simulink model "simplebc_tl"  (Simulink 7.3)
settings: Solver=FixedStepDiscrete  SolverMode=SingleTasking  StartTime=0.0  StopTime=400  FixedStep=tsample  RelTol=1e-3
PreLoadFcn:
  | if exist('tl_preloadfcn','file'), tl_preloadfcn(gcs,101); end
PostLoadFcn:
  | if exist('tl_postloadfcn','file'), tl_postloadfcn(gcs,101); end
InitFcn:
  | if exist('tlds_init','file'), tlds_init(gcs); end
StartFcn:
  | if exist('tlds_start','file'), tlds_start(gcs); end
StopFcn:
  | if exist('tlds_stop','file'), tlds_stop(gcs); end
values from neighbouring files (symbols this model uses):
  fs_max = 4000    [simplebc_mdl.m]
  fs_min = 1000    [simplebc_mdl.m]
  maxcnt_heating = 10    [simplebc_mdl.m]
  maxcnt_ign = 3    [simplebc_mdl.m]
  maxcnt_preign = 2    [simplebc_mdl.m]
  maxcnt_prev1 = 3    [simplebc_mdl.m]
  maxcnt_prev2 = 8    [simplebc_mdl.m]
  maxcnt_standby = 10    [simplebc_mdl.m]
  srinp_resptime = 2    [simplebc_mdl.m]
  srinp_testcycletime = 3    [simplebc_mdl.m]
  sroutp_resptime = 2    [simplebc_mdl.m]
  sroutp_testcycletime = 3    [simplebc_mdl.m]
  tsample = 0.1    [simplebc_mdl.m]
libraries: tllib x6, simulink x6
(part 1 of 2)
PreSaveFcn:
  | if exist('tl_presavefcn','file'), tl_presavefcn(gcs); end
settings Model: DS_PROJECTFILE=simplebc.dd  TL_MAIN_DATA={'#advcodeopt',0,'frameopt',{'mexargs',''},'logopt',{'plotinterval',0.1,'globalloggingmode',4},'date',734178.39644840278}  TL_MODEL_COMMENT=Type in your documentation HERE  TLRevision=101  Creator=alexh  LastModifiedBy=qa_user  BufferReuse=off
settings OptimizationCC: BlockReduction=off  BooleanDataType=off  InlineInvariantSignals=on  OptimizeBlockIOStorage=off  BufferReuse=off  ExpressionFolding=off  LocalBlockOutputs=off  InitFltsAndDblsToZero=on
settings DebuggingCC: SaveWithParameterizedLinksMsg=none  SignalResolutionControl=TryResolveAllWithWarning  SolverPrmCheckMsg=none  MultiTaskDSMMsg=warning  MultiTaskCondExecSysMsg=none  StrictBusMsg=ErrorLevel1
settings HardwareCC: TargetUnknown=on
settings RTWCC: IncludeERTFirstTime=on
settings GRTTargetCC: TargetFcnLib=ansi_tfl_tmw.mat  ModelReferenceCompliant=off  MatFileLogging=off

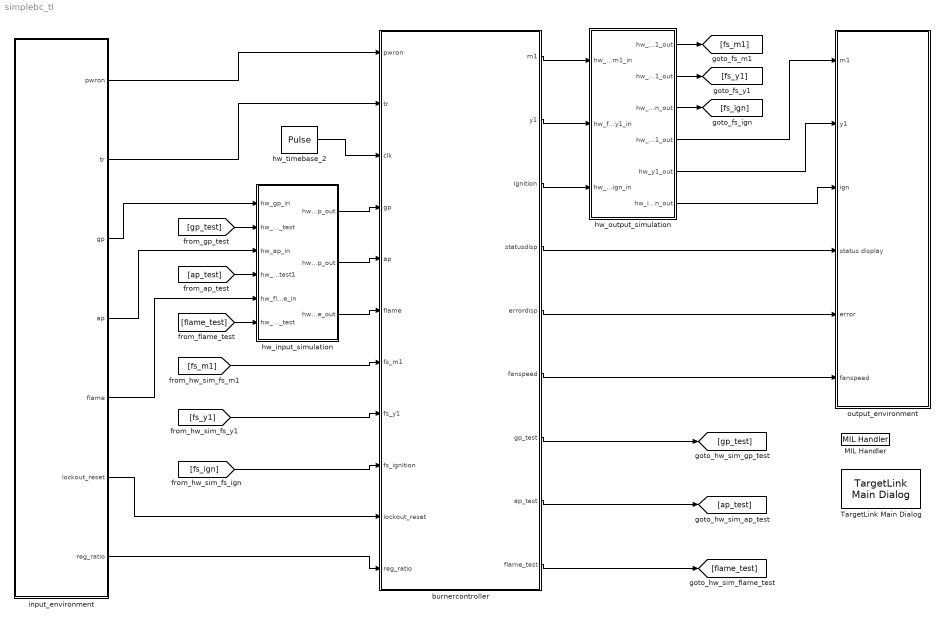
== system simplebc_tl ==
  MIL Handler : tllib/MIL Handler  data={'date',734178.39643827546}
  TargetLink Main Dialog : tllib/TargetLink Main Dialog  SystemSampleTime=-1
  burnercontroller : Subsystem  Tag=TargetLink Simulation Frame
      settings: CopyFcn=if exist('tl_copyfcn','file'), tl_copyfcn(gcbh); end  NameChangeFcn=if exist('tl_framenamechangefcn','file'), tl_framenamechangefcn(gcbh); end
      settings: OpenFcn=|
      | if exist('open_tlsubsystem','file')
      |    open_tlsubsystem(gcbh);
      | else
      |    tlsubsystem = ...
      |       find_system(gcb, ...
      |       'LookUnderMasks','on', ...
      |       'FollowLinks','on', ...
      |       'Tag','MIL Subsystem');
      |    open_system(tlsubsystem);
      | end
      mask Type: TL_SimFrame
      mask Display: disp('TargetLink\nModel-\nin-the-loop\nmode')
  hw_input_simulation : Subsystem
  hw_output_simulation : Subsystem
  hw_timebase_2 : DiscretePulseGenerator  PulseType=Time based  Amplitude=1  Period=tsample*2  PulseWidth=50  PhaseDelay=0  SampleTime=1
  input_environment : Subsystem
  output_environment : Subsystem
  wires:
  hw_input_simulation/1(hw_gp_out) -> burnercontroller/4(gp)
  input_environment/3(gp) -> hw_input_simulation/1(hw_gp_in)
  hw_input_simulation/2(hw_ap_out) -> burnercontroller/5(ap)
  hw_input_simulation/3(hw_flame_out) -> burnercontroller/6(flame)
  input_environment/4(ap) -> hw_input_simulation/3(hw_ap_in)
  input_environment/5(flame) -> hw_input_simulation/5(hw_flame_in)
  burnercontroller/8(ap_test) -> [ap_test]
  burnercontroller/9(flame_test) -> [flame_test]
  [flame_test] -> hw_input_simulation/6(hw_flame_test)
  [ap_test] -> hw_input_simulation/4(hw_ap_test1)
  [gp_test] -> hw_input_simulation/2(hw_gp_test)
  input_environment/6(lockout_reset) -> burnercontroller/10(lockout_reset)
  burnercontroller/1(m1) -> hw_output_simulation/1(hw_fs_m1_in)
  burnercontroller/2(y1) -> hw_output_simulation/2(hw_fs_y1_in)
  burnercontroller/3(ignition) -> hw_output_simulation/3(hw_fs_ign_in)
  hw_output_simulation/6(hw_ign_out) -> output_environment/3(ign)
  hw_output_simulation/3(hw_fs_ign_out) -> [fs_ign]
  hw_output_simulation/1(hw_fs_m1_out) -> [fs_m1]
  hw_output_simulation/2(hw_fs_y1_out) -> [fs_y1]
  [fs_ign] -> burnercontroller/9(fs_ignition)
  [fs_y1] -> burnercontroller/8(fs_y1)
  [fs_m1] -> burnercontroller/7(fs_m1)
  burnercontroller/4(statusdisp) -> output_environment/4(status display)
  burnercontroller/5(errordisp) -> output_environment/5(error)
  hw_output_simulation/4(hw_m1_out) -> output_environment/1(m1)
  hw_output_simulation/5(hw_y1_out) -> output_environment/2(y1)
  input_environment/7(reg_ratio) -> burnercontroller/11(reg_ratio)
  input_environment/1(pwron) -> burnercontroller/1(pwron)
  input_environment/2(tr) -> burnercontroller/2(tr)
  hw_timebase_2/1 -> burnercontroller/3(clk)
  burnercontroller/7(gp_test) -> [gp_test]
  burnercontroller/6(fanspeed) -> output_environment/6(fanspeed)

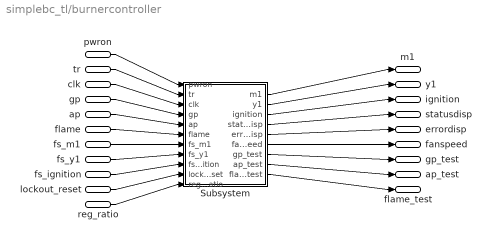
== system simplebc_tl/burnercontroller ==
  pwron : Inport  OutDataType=sfix(16)  OutScaling=2^0
  tr : Inport  Port=2  OutDataType=sfix(16)  OutScaling=2^0
  clk : Inport  Port=3  OutDataType=sfix(16)  OutScaling=2^0
  gp : Inport  Port=4  OutDataType=sfix(16)  OutScaling=2^0
  ap : Inport  Port=5  OutDataType=sfix(16)  OutScaling=2^0
  flame : Inport  Port=6  OutDataType=sfix(16)  OutScaling=2^0
  fs_m1 : Inport  Port=7  SampleTime=tsample  OutDataType=sfix(16)  OutScaling=2^0
  fs_y1 : Inport  Port=8  SampleTime=tsample  OutDataType=sfix(16)  OutScaling=2^0
  fs_ignition : Inport  Port=9  SampleTime=tsample  OutDataType=sfix(16)  OutScaling=2^0
  lockout_reset : Inport  Port=10  OutDataType=sfix(16)  OutScaling=2^0
  reg_ratio : Inport  Port=11  OutDataType=sfix(16)  OutScaling=2^0
  Subsystem : Subsystem  Tag=struct('sfcnName','burnercontroller_sf','subFunction','','srcSubsystem','')
      settings: OpenFcn=warndlg(get_param(gcb,'MaskHelp'),'Serious Warning');
      mask Type: TL_Enable
      mask Help: This subsystem keeps the TargetLink subsystem (subsystem with TargetLink blocks for production code generation), and is needed for the TargetLink simulation frame to work properly. DO NOT DELETE OR MODIFY IT!
  m1 : Outport  OutDataType=sfix(16)  OutScaling=2^0
  y1 : Outport  Port=2  OutDataType=sfix(16)  OutScaling=2^0
  ignition : Outport  Port=3  OutDataType=sfix(16)  OutScaling=2^0
  statusdisp : Outport  Port=4  OutDataType=sfix(16)  OutScaling=2^0
  errordisp : Outport  Port=5  OutDataType=sfix(16)  OutScaling=2^0
  fanspeed : Outport  Port=6  OutDataType=sfix(16)  OutScaling=2^0
  gp_test : Outport  Port=7  OutDataType=sfix(16)  OutScaling=2^0
  ap_test : Outport  Port=8  OutDataType=sfix(16)  OutScaling=2^0
  flame_test : Outport  Port=9  OutDataType=sfix(16)  OutScaling=2^0
  wires:
  pwron/1 -> Subsystem/1(pwron)
  tr/1 -> Subsystem/2(tr)
  clk/1 -> Subsystem/3(clk)
  gp/1 -> Subsystem/4(gp)
  ap/1 -> Subsystem/5(ap)
  flame/1 -> Subsystem/6(flame)
  fs_m1/1 -> Subsystem/7(fs_m1)
  fs_y1/1 -> Subsystem/8(fs_y1)
  fs_ignition/1 -> Subsystem/9(fs_ignition)
  lockout_reset/1 -> Subsystem/10(lockout_reset)
  reg_ratio/1 -> Subsystem/11(reg_ratio)
  Subsystem/1(m1) -> m1/1
  Subsystem/2(y1) -> y1/1
  Subsystem/3(ignition) -> ignition/1
  Subsystem/4(statusdisp) -> statusdisp/1
  Subsystem/5(errordisp) -> errordisp/1
  Subsystem/6(fanspeed) -> fanspeed/1
  Subsystem/7(gp_test) -> gp_test/1
  Subsystem/8(ap_test) -> ap_test/1
  Subsystem/9(flame_test) -> flame_test/1

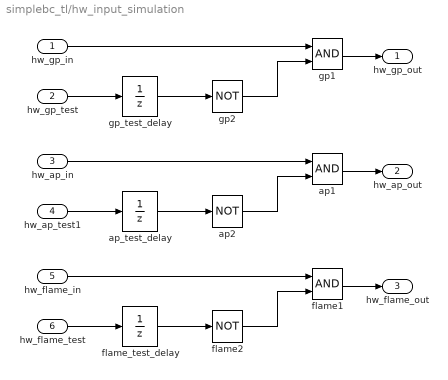
== system simplebc_tl/hw_input_simulation ==
  hw_gp_in : Inport  OutDataType=sfix(16)  OutScaling=2^0
  hw_gp_test : Inport  Port=2  OutDataType=sfix(16)  OutScaling=2^0
  hw_ap_in : Inport  Port=3  OutDataType=sfix(16)  OutScaling=2^0
  hw_ap_test1 : Inport  Port=4  OutDataType=sfix(16)  OutScaling=2^0
  hw_flame_in : Inport  Port=5  OutDataType=sfix(16)  OutScaling=2^0
  hw_flame_test : Inport  Port=6  OutDataType=sfix(16)  OutScaling=2^0
  ap1 : Logic
  ap2 : Logic  Operator=NOT  Inputs=1
  ap_test_delay : UnitDelay  SampleTime=tsample*2
  flame1 : Logic
  flame2 : Logic  Operator=NOT  Inputs=1
  flame_test_delay : UnitDelay  SampleTime=tsample*2
  gp1 : Logic
  gp2 : Logic  Operator=NOT  Inputs=1
  gp_test_delay : UnitDelay  SampleTime=tsample*2
  hw_gp_out : Outport  OutDataType=sfix(16)  OutScaling=2^0
  hw_ap_out : Outport  Port=2  OutDataType=sfix(16)  OutScaling=2^0
  hw_flame_out : Outport  Port=3  OutDataType=sfix(16)  OutScaling=2^0
  wires:
  gp2/1 -> gp1/2
  gp_test_delay/1 -> gp2/1
  hw_gp_test/1 -> gp_test_delay/1
  hw_gp_in/1 -> gp1/1
  gp1/1 -> hw_gp_out/1
  ap2/1 -> ap1/2
  ap_test_delay/1 -> ap2/1
  hw_ap_test1/1 -> ap_test_delay/1
  hw_ap_in/1 -> ap1/1
  ap1/1 -> hw_ap_out/1
  flame2/1 -> flame1/2
  flame_test_delay/1 -> flame2/1
  hw_flame_test/1 -> flame_test_delay/1
  hw_flame_in/1 -> flame1/1
  flame1/1 -> hw_flame_out/1

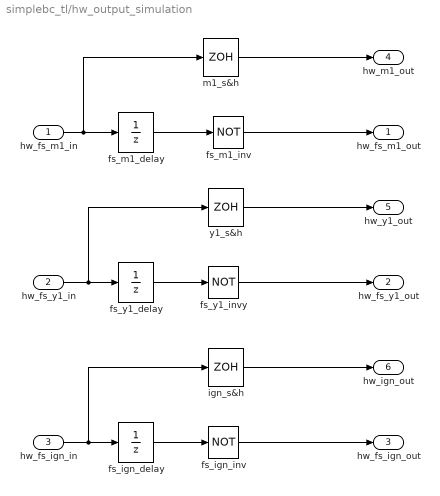
== system simplebc_tl/hw_output_simulation ==
  hw_fs_m1_in : Inport  OutDataType=sfix(16)  OutScaling=2^0
  hw_fs_y1_in : Inport  Port=2  OutDataType=sfix(16)  OutScaling=2^0
  hw_fs_ign_in : Inport  Port=3  OutDataType=sfix(16)  OutScaling=2^0
  fs_ign_delay : UnitDelay  SampleTime=tsample*2
  fs_ign_inv : Logic  Operator=NOT  Inputs=1
  fs_m1_delay : UnitDelay  SampleTime=tsample*2
  fs_m1_inv : Logic  Operator=NOT  Inputs=1
  fs_y1_delay : UnitDelay  SampleTime=tsample*2
  fs_y1_invy : Logic  Operator=NOT  Inputs=1
  ign_s&h : ZeroOrderHold  SampleTime=tsample*(sroutp_testcycletime+sroutp_resptime)
  m1_s&h : ZeroOrderHold  SampleTime=tsample*(sroutp_testcycletime+sroutp_resptime)
  y1_s&h : ZeroOrderHold  SampleTime=tsample*(sroutp_testcycletime+sroutp_resptime)
  hw_fs_m1_out : Outport  OutDataType=sfix(16)  OutScaling=2^0
  hw_fs_y1_out : Outport  Port=2  OutDataType=sfix(16)  OutScaling=2^0
  hw_fs_ign_out : Outport  Port=3  OutDataType=sfix(16)  OutScaling=2^0
  hw_m1_out : Outport  Port=4  OutDataType=sfix(16)  OutScaling=2^0
  hw_y1_out : Outport  Port=5  OutDataType=sfix(16)  OutScaling=2^0
  hw_ign_out : Outport  Port=6  OutDataType=sfix(16)  OutScaling=2^0
  wires:
  fs_m1_inv/1 -> hw_fs_m1_out/1
  hw_fs_m1_in/1 -> fs_m1_delay/1, m1_s&h/1
  m1_s&h/1 -> hw_m1_out/1
  fs_y1_delay/1 -> fs_y1_invy/1
  fs_y1_invy/1 -> hw_fs_y1_out/1
  hw_fs_y1_in/1 -> fs_y1_delay/1, y1_s&h/1
  y1_s&h/1 -> hw_y1_out/1
  fs_ign_delay/1 -> fs_ign_inv/1
  fs_ign_inv/1 -> hw_fs_ign_out/1
  hw_fs_ign_in/1 -> fs_ign_delay/1, ign_s&h/1
  ign_s&h/1 -> hw_ign_out/1
  fs_m1_delay/1 -> fs_m1_inv/1

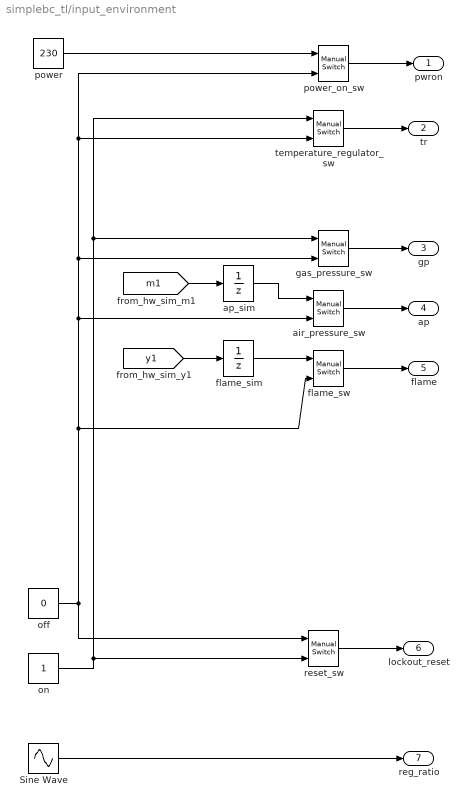
== system simplebc_tl/input_environment ==
  Sine Wave : Sin  Amplitude=50  Bias=50  Frequency=0.01  Phase=0  Samples=10  SampleTime=0  Offset=0
  air_pressure_sw : simulink/Signal Routing/Manual Switch  SystemSampleTime=-1  sw=1  action=0  varsize=off
  ap_sim : UnitDelay  SampleTime=tsample*10
  flame_sim : UnitDelay  SampleTime=tsample*10
  flame_sw : simulink/Signal Routing/Manual Switch  SystemSampleTime=-1  sw=1  action=0  varsize=off
  gas_pressure_sw : simulink/Signal Routing/Manual Switch  SystemSampleTime=-1  sw=1  action=0  varsize=off
  off : Constant  Value=0  OutDataType=sfix(16)  OutScaling=2^0
  on : Constant  OutDataType=sfix(16)  OutScaling=2^0
  power : Constant  Value=230  OutDataType=sfix(16)  OutScaling=2^0
  power_on_sw : simulink/Signal Routing/Manual Switch  SystemSampleTime=-1  sw=1  action=0  varsize=off
  reset_sw : simulink/Signal Routing/Manual Switch  SystemSampleTime=-1  sw=1  action=0  varsize=off
  temperature_regulator_sw : simulink/Signal Routing/Manual Switch  SystemSampleTime=-1  sw=1  action=0  varsize=off
  pwron : Outport  OutDataType=sfix(16)  OutScaling=2^0
  tr : Outport  Port=2  OutDataType=sfix(16)  OutScaling=2^0
  gp : Outport  Port=3  OutDataType=sfix(16)  OutScaling=2^0
  ap : Outport  Port=4  OutDataType=sfix(16)  OutScaling=2^0
  flame : Outport  Port=5  OutDataType=sfix(16)  OutScaling=2^0
  lockout_reset : Outport  Port=6  OutDataType=sfix(16)  OutScaling=2^0
  reg_ratio : Outport  Port=7  OutDataType=sfix(16)  OutScaling=2^0
  wires:
  flame_sim/1 -> flame_sw/1
  ap_sim/1 -> air_pressure_sw/1
  [m1] -> ap_sim/1
  [y1] -> flame_sim/1
  on/1 -> temperature_regulator_sw/1, gas_pressure_sw/1, reset_sw/2
  off/1 -> power_on_sw/2, temperature_regulator_sw/2, gas_pressure_sw/2, air_pressure_sw/2, flame_sw/2, reset_sw/1
  power/1 -> power_on_sw/1
  power_on_sw/1 -> pwron/1
  temperature_regulator_sw/1 -> tr/1
  gas_pressure_sw/1 -> gp/1
  air_pressure_sw/1 -> ap/1
  flame_sw/1 -> flame/1
  reset_sw/1 -> lockout_reset/1
  Sine Wave/1 -> reg_ratio/1

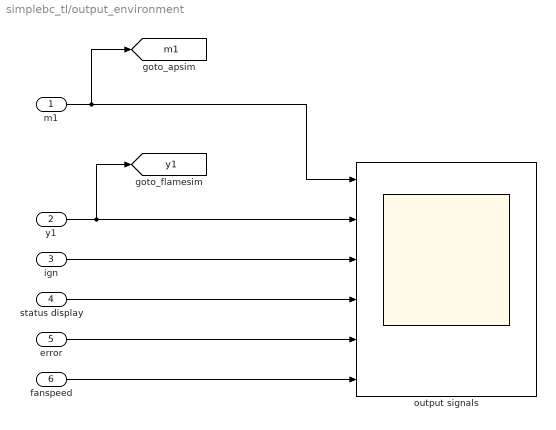
== system simplebc_tl/output_environment ==
  m1 : Inport  OutDataType=sfix(16)  OutScaling=2^0
  y1 : Inport  Port=2  OutDataType=sfix(16)  OutScaling=2^0
  ign : Inport  Port=3  OutDataType=sfix(16)  OutScaling=2^0
  status display : Inport  Port=4  OutDataType=sfix(16)  OutScaling=2^0
  error : Inport  Port=5  OutDataType=sfix(16)  OutScaling=2^0
  fanspeed : Inport  Port=6  OutDataType=sfix(16)  OutScaling=2^0
  output signals : Scope  NumInputPorts=6
      settings: TimeRange=400  YMin=0~0~0~0~0~0  YMax=1.5~1.5~1.5~8~1.5~8000
  tag scope: m1=global, y1=global
  wires:
  y1/1 -> [y1], output signals/2
  m1/1 -> [m1], output signals/1
  ign/1 -> output signals/3
  status display/1 -> output signals/4
  error/1 -> output signals/5
  fanspeed/1 -> output signals/6

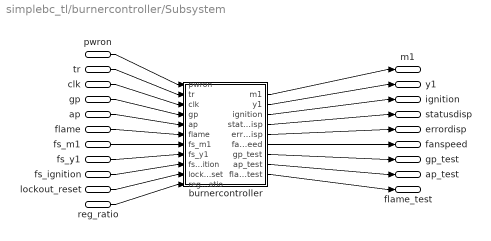
== system simplebc_tl/burnercontroller/Subsystem ==
  pwron : Inport  OutDataType=sfix(16)  OutScaling=2^0
  tr : Inport  Port=2  OutDataType=sfix(16)  OutScaling=2^0
  clk : Inport  Port=3  OutDataType=sfix(16)  OutScaling=2^0
  gp : Inport  Port=4  OutDataType=sfix(16)  OutScaling=2^0
  ap : Inport  Port=5  OutDataType=sfix(16)  OutScaling=2^0
  flame : Inport  Port=6  OutDataType=sfix(16)  OutScaling=2^0
  fs_m1 : Inport  Port=7  SampleTime=tsample  OutDataType=sfix(16)  OutScaling=2^0
  fs_y1 : Inport  Port=8  SampleTime=tsample  OutDataType=sfix(16)  OutScaling=2^0
  fs_ignition : Inport  Port=9  SampleTime=tsample  OutDataType=sfix(16)  OutScaling=2^0
  lockout_reset : Inport  Port=10  OutDataType=sfix(16)  OutScaling=2^0
  reg_ratio : Inport  Port=11  OutDataType=sfix(16)  OutScaling=2^0
  burnercontroller : Subsystem  Tag=MIL Subsystem  Description=a
      settings: CopyFcn=if exist('tl_copyfcn','file'), tl_copyfcn(gcbh); end  NameChangeFcn=if exist('tl_namechangefcn','file'), tl_namechangefcn(gcbh); end  DestroyFcn=if exist('update_tl_main_dlg','file'), update_tl_main_dlg('TL_subs_display'); end
      mask Display: disp('TargetLink Subsystem')
  m1 : Outport  OutDataType=sfix(16)  OutScaling=2^0
  y1 : Outport  Port=2  OutDataType=sfix(16)  OutScaling=2^0
  ignition : Outport  Port=3  OutDataType=sfix(16)  OutScaling=2^0
  statusdisp : Outport  Port=4  OutDataType=sfix(16)  OutScaling=2^0
  errordisp : Outport  Port=5  OutDataType=sfix(16)  OutScaling=2^0
  fanspeed : Outport  Port=6  OutDataType=sfix(16)  OutScaling=2^0
  gp_test : Outport  Port=7  OutDataType=sfix(16)  OutScaling=2^0
  ap_test : Outport  Port=8  OutDataType=sfix(16)  OutScaling=2^0
  flame_test : Outport  Port=9  OutDataType=sfix(16)  OutScaling=2^0
  wires:
  pwron/1 -> burnercontroller/1(pwron)
  tr/1 -> burnercontroller/2(tr)
  clk/1 -> burnercontroller/3(clk)
  gp/1 -> burnercontroller/4(gp)
  ap/1 -> burnercontroller/5(ap)
  flame/1 -> burnercontroller/6(flame)
  fs_m1/1 -> burnercontroller/7(fs_m1)
  fs_y1/1 -> burnercontroller/8(fs_y1)
  fs_ignition/1 -> burnercontroller/9(fs_ignition)
  lockout_reset/1 -> burnercontroller/10(lockout_reset)
  reg_ratio/1 -> burnercontroller/11(reg_ratio)
  burnercontroller/1(m1) -> m1/1
  burnercontroller/2(y1) -> y1/1
  burnercontroller/3(ignition) -> ignition/1
  burnercontroller/4(statusdisp) -> statusdisp/1
  burnercontroller/5(errordisp) -> errordisp/1
  burnercontroller/6(fanspeed) -> fanspeed/1
  burnercontroller/7(gp_test) -> gp_test/1
  burnercontroller/8(ap_test) -> ap_test/1
  burnercontroller/9(flame_test) -> flame_test/1

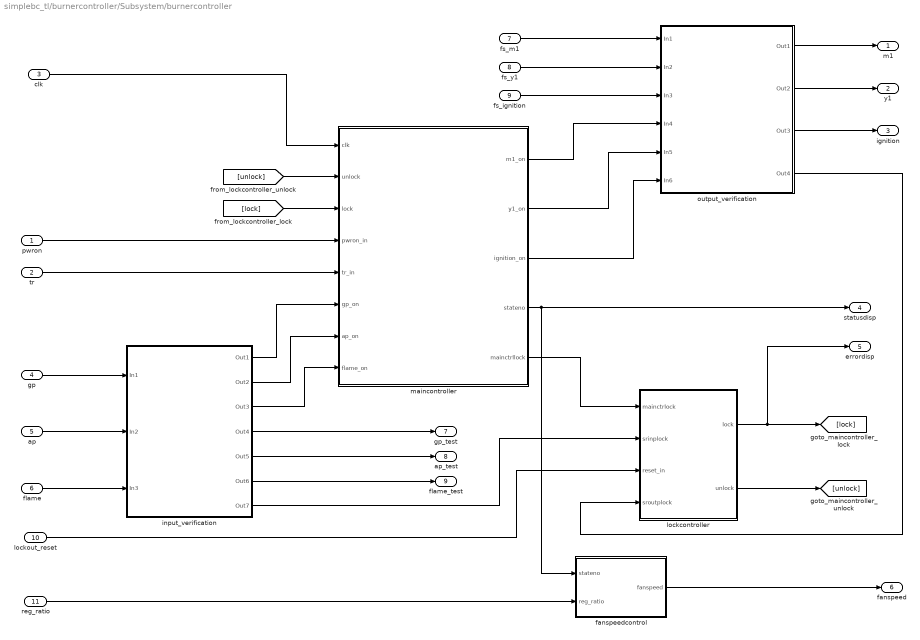
== system simplebc_tl/burnercontroller/Subsystem/burnercontroller ==
  pwron : Inport  PortDimensions=1  OutDataType=sfix(16)  OutScaling=2^0  mask(TL_Inport){data={'logdata',{'plotchannels',[]},'output',{'type','UInt8'},'date',734178.39643809025}}
      settings: DeleteFcn=if exist('delete_tlblock','file')==2,delete_tlblock(gcbh);end  OpenFcn=if exist('tl_open_blockdlg','file')==2,tl_open_blockdlg(gcbh);else,open_system(gcbh,'parameter');end
      settings: CopyFcn=|
      | if exist('tl_reset_reviewflag','file')==2
      |     tl_reset_reviewflag(gcbh);
      | end
      | if exist('tl_check_ports','file')
      |     tl_check_ports(gcbh);
      | end
      settings: NameChangeFcn=|
      | if exist('rename_tlblock','file')==2,rename_tlblock(gcbh);end
      | if exist('tl_check_ports','file'), tl_check_ports(gcbh); end
      mask Help: eval(['if exist(''tl_online_help'',''file'') == 2, tl_online_help(''Topic'',''TL_Inport''),else, web([''jar:file:///'',matlabroot,''/help/toolbox/simulink/help.jar!/slref/' lower(get_param(gcbh,'Blocktype')) '.html''], ''-helpbrowser''),end'])
      mask Display: plot([0.2 0.35 NaN 0.65 0.8],[0 1 NaN 0 1]);
  tr : Inport  Port=2  PortDimensions=1  OutDataType=sfix(16)  OutScaling=2^0  mask(TL_Inport){data={'logdata',{'plotchannels',[]},'output',{'type','Bool'},'date',734178.39643773146}}
      settings: DeleteFcn=if exist('delete_tlblock','file')==2,delete_tlblock(gcbh);end  OpenFcn=if exist('tl_open_blockdlg','file')==2,tl_open_blockdlg(gcbh);else,open_system(gcbh,'parameter');end
      settings: CopyFcn=|
      | if exist('tl_reset_reviewflag','file')==2
      |     tl_reset_reviewflag(gcbh);
      | end
      | if exist('tl_check_ports','file')
      |     tl_check_ports(gcbh);
      | end
      settings: NameChangeFcn=|
      | if exist('rename_tlblock','file')==2,rename_tlblock(gcbh);end
      | if exist('tl_check_ports','file'), tl_check_ports(gcbh); end
      mask Help: eval(['if exist(''tl_online_help'',''file'') == 2, tl_online_help(''Topic'',''TL_Inport''),else, web([''jar:file:///'',matlabroot,''/help/toolbox/simulink/help.jar!/slref/' lower(get_param(gcbh,'Blocktype')) '.html''], ''-helpbrowser''),end'])
      mask Display: plot([0.2 0.35 NaN 0.65 0.8],[0 1 NaN 0 1]);
  clk : Inport  Port=3  PortDimensions=1  OutDataType=sfix(16)  OutScaling=2^0  mask(TL_Inport){data={'logdata',{'plotchannels',[]},'date',734178.39643718745}}
      settings: DeleteFcn=if exist('delete_tlblock','file')==2,delete_tlblock(gcbh);end  OpenFcn=if exist('tl_open_blockdlg','file')==2,tl_open_blockdlg(gcbh);else,open_system(gcbh,'parameter');end
      settings: CopyFcn=|
      | if exist('tl_reset_reviewflag','file')==2
      |     tl_reset_reviewflag(gcbh);
      | end
      | if exist('tl_check_ports','file')
      |     tl_check_ports(gcbh);
      | end
      settings: NameChangeFcn=|
      | if exist('rename_tlblock','file')==2,rename_tlblock(gcbh);end
      | if exist('tl_check_ports','file'), tl_check_ports(gcbh); end
      mask Help: eval(['if exist(''tl_online_help'',''file'') == 2, tl_online_help(''Topic'',''TL_Inport''),else, web([''jar:file:///'',matlabroot,''/help/toolbox/simulink/help.jar!/slref/' lower(get_param(gcbh,'Blocktype')) '.html''], ''-helpbrowser''),end'])
      mask Display: plot([0.2 0.35 NaN 0.65 0.8],[0 1 NaN 0 1]);
  gp : Inport  Port=4  PortDimensions=1  OutDataType=sfix(16)  OutScaling=2^0  mask(TL_Inport){data={'logdata',{'plotchannels',[]},'output',{'type','Bool'},'date',734178.39643682865}}
      settings: DeleteFcn=if exist('delete_tlblock','file')==2,delete_tlblock(gcbh);end  OpenFcn=if exist('tl_open_blockdlg','file')==2,tl_open_blockdlg(gcbh);else,open_system(gcbh,'parameter');end
      settings: CopyFcn=|
      | if exist('tl_reset_reviewflag','file')==2
      |     tl_reset_reviewflag(gcbh);
      | end
      | if exist('tl_check_ports','file')
      |     tl_check_ports(gcbh);
      | end
      settings: NameChangeFcn=|
      | if exist('rename_tlblock','file')==2,rename_tlblock(gcbh);end
      | if exist('tl_check_ports','file'), tl_check_ports(gcbh); end
      mask Help: eval(['if exist(''tl_online_help'',''file'') == 2, tl_online_help(''Topic'',''TL_Inport''),else, web([''jar:file:///'',matlabroot,''/help/toolbox/simulink/help.jar!/slref/' lower(get_param(gcbh,'Blocktype')) '.html''], ''-helpbrowser''),end'])
      mask Display: plot([0.2 0.35 NaN 0.65 0.8],[0 1 NaN 0 1]);
  ap : Inport  Port=5  PortDimensions=1  OutDataType=sfix(16)  OutScaling=2^0  mask(TL_Inport){data={'logdata',{'plotchannels',[]},'output',{'type','Bool'},'date',734178.39643646986}}
      settings: DeleteFcn=if exist('delete_tlblock','file')==2,delete_tlblock(gcbh);end  OpenFcn=if exist('tl_open_blockdlg','file')==2,tl_open_blockdlg(gcbh);else,open_system(gcbh,'parameter');end
      settings: CopyFcn=|
      | if exist('tl_reset_reviewflag','file')==2
      |     tl_reset_reviewflag(gcbh);
      | end
      | if exist('tl_check_ports','file')
      |     tl_check_ports(gcbh);
      | end
      settings: NameChangeFcn=|
      | if exist('rename_tlblock','file')==2,rename_tlblock(gcbh);end
      | if exist('tl_check_ports','file'), tl_check_ports(gcbh); end
      mask Help: eval(['if exist(''tl_online_help'',''file'') == 2, tl_online_help(''Topic'',''TL_Inport''),else, web([''jar:file:///'',matlabroot,''/help/toolbox/simulink/help.jar!/slref/' lower(get_param(gcbh,'Blocktype')) '.html''], ''-helpbrowser''),end'])
      mask Display: plot([0.2 0.35 NaN 0.65 0.8],[0 1 NaN 0 1]);
  flame : Inport  Port=6  PortDimensions=1  OutDataType=sfix(16)  OutScaling=2^0  mask(TL_Inport){data={'logdata',{'plotchannels',[]},'output',{'type','Bool'},'date',734178.39643592597}}
      settings: DeleteFcn=if exist('delete_tlblock','file')==2,delete_tlblock(gcbh);end  OpenFcn=if exist('tl_open_blockdlg','file')==2,tl_open_blockdlg(gcbh);else,open_system(gcbh,'parameter');end
      settings: CopyFcn=|
      | if exist('tl_reset_reviewflag','file')==2
      |     tl_reset_reviewflag(gcbh);
      | end
      | if exist('tl_check_ports','file')
      |     tl_check_ports(gcbh);
      | end
      settings: NameChangeFcn=|
      | if exist('rename_tlblock','file')==2,rename_tlblock(gcbh);end
      | if exist('tl_check_ports','file'), tl_check_ports(gcbh); end
      mask Help: eval(['if exist(''tl_online_help'',''file'') == 2, tl_online_help(''Topic'',''TL_Inport''),else, web([''jar:file:///'',matlabroot,''/help/toolbox/simulink/help.jar!/slref/' lower(get_param(gcbh,'Blocktype')) '.html''], ''-helpbrowser''),end'])
      mask Display: plot([0.2 0.35 NaN 0.65 0.8],[0 1 NaN 0 1]);
  fs_m1 : Inport  Port=7  PortDimensions=1  SampleTime=tsample  OutDataType=sfix(16)  OutScaling=2^0  mask(TL_Inport){data={'logdata',{'plotchannels',[]},'output',{'type','Bool'},'date',734178.39643555554}}
      settings: DeleteFcn=if exist('delete_tlblock','file')==2,delete_tlblock(gcbh);end  OpenFcn=if exist('tl_open_blockdlg','file')==2,tl_open_blockdlg(gcbh);else,open_system(gcbh,'parameter');end
      settings: CopyFcn=|
      | if exist('tl_reset_reviewflag','file')==2
      |     tl_reset_reviewflag(gcbh);
      | end
      | if exist('tl_check_ports','file')
      |     tl_check_ports(gcbh);
      | end
      settings: NameChangeFcn=|
      | if exist('rename_tlblock','file')==2,rename_tlblock(gcbh);end
      | if exist('tl_check_ports','file'), tl_check_ports(gcbh); end
      mask Help: eval(['if exist(''tl_online_help'',''file'') == 2, tl_online_help(''Topic'',''TL_Inport''),else, web([''jar:file:///'',matlabroot,''/help/toolbox/simulink/help.jar!/slref/' lower(get_param(gcbh,'Blocktype')) '.html''], ''-helpbrowser''),end'])
      mask Display: plot([0.2 0.35 NaN 0.65 0.8],[0 1 NaN 0 1]);
  fs_y1 : Inport  Port=8  PortDimensions=1  SampleTime=tsample  OutDataType=sfix(16)  OutScaling=2^0  mask(TL_Inport){data={'logdata',{'plotchannels',[]},'output',{'type','Bool'},'date',734178.39643519674}}
      settings: DeleteFcn=if exist('delete_tlblock','file')==2,delete_tlblock(gcbh);end  OpenFcn=if exist('tl_open_blockdlg','file')==2,tl_open_blockdlg(gcbh);else,open_system(gcbh,'parameter');end
      settings: CopyFcn=|
      | if exist('tl_reset_reviewflag','file')==2
      |     tl_reset_reviewflag(gcbh);
      | end
      | if exist('tl_check_ports','file')
      |     tl_check_ports(gcbh);
      | end
      settings: NameChangeFcn=|
      | if exist('rename_tlblock','file')==2,rename_tlblock(gcbh);end
      | if exist('tl_check_ports','file'), tl_check_ports(gcbh); end
      mask Help: eval(['if exist(''tl_online_help'',''file'') == 2, tl_online_help(''Topic'',''TL_Inport''),else, web([''jar:file:///'',matlabroot,''/help/toolbox/simulink/help.jar!/slref/' lower(get_param(gcbh,'Blocktype')) '.html''], ''-helpbrowser''),end'])
      mask Display: plot([0.2 0.35 NaN 0.65 0.8],[0 1 NaN 0 1]);
  fs_ignition : Inport  Port=9  PortDimensions=1  SampleTime=tsample  OutDataType=sfix(16)  OutScaling=2^0  mask(TL_Inport){data={'logdata',{'plotchannels',[]},'output',{'type','Bool'},'date',734178.39643465274}}
      settings: DeleteFcn=if exist('delete_tlblock','file')==2,delete_tlblock(gcbh);end  OpenFcn=if exist('tl_open_blockdlg','file')==2,tl_open_blockdlg(gcbh);else,open_system(gcbh,'parameter');end
      settings: CopyFcn=|
      | if exist('tl_reset_reviewflag','file')==2
      |     tl_reset_reviewflag(gcbh);
      | end
      | if exist('tl_check_ports','file')
      |     tl_check_ports(gcbh);
      | end
      settings: NameChangeFcn=|
      | if exist('rename_tlblock','file')==2,rename_tlblock(gcbh);end
      | if exist('tl_check_ports','file'), tl_check_ports(gcbh); end
      mask Help: eval(['if exist(''tl_online_help'',''file'') == 2, tl_online_help(''Topic'',''TL_Inport''),else, web([''jar:file:///'',matlabroot,''/help/toolbox/simulink/help.jar!/slref/' lower(get_param(gcbh,'Blocktype')) '.html''], ''-helpbrowser''),end'])
      mask Display: plot([0.2 0.35 NaN 0.65 0.8],[0 1 NaN 0 1]);
  lockout_reset : Inport  Port=10  PortDimensions=1  OutDataType=sfix(16)  OutScaling=2^0  mask(TL_Inport){data={'logdata',{'plotchannels',[]},'output',{'type','Bool'},'date',734178.39643429394}}
      settings: DeleteFcn=if exist('delete_tlblock','file')==2,delete_tlblock(gcbh);end  OpenFcn=if exist('tl_open_blockdlg','file')==2,tl_open_blockdlg(gcbh);else,open_system(gcbh,'parameter');end
      settings: CopyFcn=|
      | if exist('tl_reset_reviewflag','file')==2
      |     tl_reset_reviewflag(gcbh);
      | end
      | if exist('tl_check_ports','file')
      |     tl_check_ports(gcbh);
      | end
      settings: NameChangeFcn=|
      | if exist('rename_tlblock','file')==2,rename_tlblock(gcbh);end
      | if exist('tl_check_ports','file'), tl_check_ports(gcbh); end
      mask Help: eval(['if exist(''tl_online_help'',''file'') == 2, tl_online_help(''Topic'',''TL_Inport''),else, web([''jar:file:///'',matlabroot,''/help/toolbox/simulink/help.jar!/slref/' lower(get_param(gcbh,'Blocktype')) '.html''], ''-helpbrowser''),end'])
      mask Display: plot([0.2 0.35 NaN 0.65 0.8],[0 1 NaN 0 1]);
  reg_ratio : Inport  Port=11  PortDimensions=1  OutDataType=sfix(16)  OutScaling=2^0  mask(TL_Inport){data={'logdata',{'plotchannels',[]},'date',734178.39643375005}}
      settings: DeleteFcn=if exist('delete_tlblock','file')==2,delete_tlblock(gcbh);end  OpenFcn=if exist('tl_open_blockdlg','file')==2,tl_open_blockdlg(gcbh);else,open_system(gcbh,'parameter');end
      settings: CopyFcn=|
      | if exist('tl_reset_reviewflag','file')==2
      |     tl_reset_reviewflag(gcbh);
      | end
      | if exist('tl_check_ports','file')
      |     tl_check_ports(gcbh);
      | end
      settings: NameChangeFcn=|
      | if exist('rename_tlblock','file')==2,rename_tlblock(gcbh);end
      | if exist('tl_check_ports','file'), tl_check_ports(gcbh); end
      mask Help: eval(['if exist(''tl_online_help'',''file'') == 2, tl_online_help(''Topic'',''TL_Inport''),else, web([''jar:file:///'',matlabroot,''/help/toolbox/simulink/help.jar!/slref/' lower(get_param(gcbh,'Blocktype')) '.html''], ''-helpbrowser''),end'])
      mask Display: plot([0.2 0.35 NaN 0.65 0.8],[0 1 NaN 0 1]);
  fanspeedcontrol : Subsystem  TreatAsAtomicUnit=on
  input_verification : Subsystem  TreatAsAtomicUnit=on
  lockcontroller : Subsystem
  maincontroller : Subsystem  TreatAsAtomicUnit=on
  output_verification : Subsystem  TreatAsAtomicUnit=on
  m1 : Outport  PortDimensions=1  OutDataType=sfix(16)  OutScaling=2^0  mask(TL_Outport){data={'logdata',{'plotchannels',[]},'date',734178.39642506943}}
      settings: DeleteFcn=if exist('delete_tlblock','file')==2,delete_tlblock(gcbh);end  OpenFcn=if exist('tl_open_blockdlg','file')==2,tl_open_blockdlg(gcbh);else,open_system(gcbh,'parameter');end
      settings: CopyFcn=|
      | if exist('tl_reset_reviewflag','file')==2
      |     tl_reset_reviewflag(gcbh);
      | end
      | if exist('tl_check_ports','file')
      |     tl_check_ports(gcbh);
      | end
      settings: NameChangeFcn=|
      | if exist('rename_tlblock','file')==2,rename_tlblock(gcbh);end
      | if exist('tl_check_ports','file'), tl_check_ports(gcbh); end
      mask Help: eval(['if exist(''tl_online_help'',''file'') == 2, tl_online_help(''Topic'',''TL_Outport''),else, web([''jar:file:///'',matlabroot,''/help/toolbox/simulink/help.jar!/slref/' lower(get_param(gcbh,'Blocktype')) '.html''], ''-helpbrowser''),end'])
      mask Display: plot([0.2 0.35 NaN 0.65 0.8],[0 1 NaN 0 1]);
  y1 : Outport  Port=2  PortDimensions=1  OutDataType=sfix(16)  OutScaling=2^0  mask(TL_Outport){data={'logdata',{'plotchannels',[]},'date',734178.39642452542}}
      settings: DeleteFcn=if exist('delete_tlblock','file')==2,delete_tlblock(gcbh);end  OpenFcn=if exist('tl_open_blockdlg','file')==2,tl_open_blockdlg(gcbh);else,open_system(gcbh,'parameter');end
      settings: CopyFcn=|
      | if exist('tl_reset_reviewflag','file')==2
      |     tl_reset_reviewflag(gcbh);
      | end
      | if exist('tl_check_ports','file')
      |     tl_check_ports(gcbh);
      | end
      settings: NameChangeFcn=|
      | if exist('rename_tlblock','file')==2,rename_tlblock(gcbh);end
      | if exist('tl_check_ports','file'), tl_check_ports(gcbh); end
      mask Help: eval(['if exist(''tl_online_help'',''file'') == 2, tl_online_help(''Topic'',''TL_Outport''),else, web([''jar:file:///'',matlabroot,''/help/toolbox/simulink/help.jar!/slref/' lower(get_param(gcbh,'Blocktype')) '.html''], ''-helpbrowser''),end'])
      mask Display: plot([0.2 0.35 NaN 0.65 0.8],[0 1 NaN 0 1]);
  ignition : Outport  Port=3  PortDimensions=1  OutDataType=sfix(16)  OutScaling=2^0  mask(TL_Outport){data={'logdata',{'plotchannels',[]},'output',{'type','Bool'},'date',734178.39642416663}}
      settings: DeleteFcn=if exist('delete_tlblock','file')==2,delete_tlblock(gcbh);end  OpenFcn=if exist('tl_open_blockdlg','file')==2,tl_open_blockdlg(gcbh);else,open_system(gcbh,'parameter');end
      settings: CopyFcn=|
      | if exist('tl_reset_reviewflag','file')==2
      |     tl_reset_reviewflag(gcbh);
      | end
      | if exist('tl_check_ports','file')
      |     tl_check_ports(gcbh);
      | end
      settings: NameChangeFcn=|
      | if exist('rename_tlblock','file')==2,rename_tlblock(gcbh);end
      | if exist('tl_check_ports','file'), tl_check_ports(gcbh); end
      mask Help: eval(['if exist(''tl_online_help'',''file'') == 2, tl_online_help(''Topic'',''TL_Outport''),else, web([''jar:file:///'',matlabroot,''/help/toolbox/simulink/help.jar!/slref/' lower(get_param(gcbh,'Blocktype')) '.html''], ''-helpbrowser''),end'])
      mask Display: plot([0.2 0.35 NaN 0.65 0.8],[0 1 NaN 0 1]);
  statusdisp : Outport  Port=4  PortDimensions=1  OutDataType=sfix(16)  OutScaling=2^0  mask(TL_Outport){data={'logdata',{'plotchannels',[]},'date',734178.39642362273}}
      settings: DeleteFcn=if exist('delete_tlblock','file')==2,delete_tlblock(gcbh);end  OpenFcn=if exist('tl_open_blockdlg','file')==2,tl_open_blockdlg(gcbh);else,open_system(gcbh,'parameter');end
      settings: CopyFcn=|
      | if exist('tl_reset_reviewflag','file')==2
      |     tl_reset_reviewflag(gcbh);
      | end
      | if exist('tl_check_ports','file')
      |     tl_check_ports(gcbh);
      | end
      settings: NameChangeFcn=|
      | if exist('rename_tlblock','file')==2,rename_tlblock(gcbh);end
      | if exist('tl_check_ports','file'), tl_check_ports(gcbh); end
      mask Help: eval(['if exist(''tl_online_help'',''file'') == 2, tl_online_help(''Topic'',''TL_Outport''),else, web([''jar:file:///'',matlabroot,''/help/toolbox/simulink/help.jar!/slref/' lower(get_param(gcbh,'Blocktype')) '.html''], ''-helpbrowser''),end'])
      mask Display: plot([0.2 0.35 NaN 0.65 0.8],[0 1 NaN 0 1]);
  errordisp : Outport  Port=5  PortDimensions=1  OutDataType=sfix(16)  OutScaling=2^0  mask(TL_Outport){data={'logdata',{'plotchannels',[]},'date',734178.39642326394}}
      settings: DeleteFcn=if exist('delete_tlblock','file')==2,delete_tlblock(gcbh);end  OpenFcn=if exist('tl_open_blockdlg','file')==2,tl_open_blockdlg(gcbh);else,open_system(gcbh,'parameter');end
      settings: CopyFcn=|
      | if exist('tl_reset_reviewflag','file')==2
      |     tl_reset_reviewflag(gcbh);
      | end
      | if exist('tl_check_ports','file')
      |     tl_check_ports(gcbh);
      | end
      settings: NameChangeFcn=|
      | if exist('rename_tlblock','file')==2,rename_tlblock(gcbh);end
      | if exist('tl_check_ports','file'), tl_check_ports(gcbh); end
      mask Help: eval(['if exist(''tl_online_help'',''file'') == 2, tl_online_help(''Topic'',''TL_Outport''),else, web([''jar:file:///'',matlabroot,''/help/toolbox/simulink/help.jar!/slref/' lower(get_param(gcbh,'Blocktype')) '.html''], ''-helpbrowser''),end'])
      mask Display: plot([0.2 0.35 NaN 0.65 0.8],[0 1 NaN 0 1]);
  fanspeed : Outport  Port=6  PortDimensions=1  OutDataType=sfix(16)  OutScaling=2^0  mask(TL_Outport){data={'logdata',{'plotchannels',[]},'date',734178.39642271993}}
      settings: DeleteFcn=if exist('delete_tlblock','file')==2,delete_tlblock(gcbh);end  OpenFcn=if exist('tl_open_blockdlg','file')==2,tl_open_blockdlg(gcbh);else,open_system(gcbh,'parameter');end
      settings: CopyFcn=|
      | if exist('tl_reset_reviewflag','file')==2
      |     tl_reset_reviewflag(gcbh);
      | end
      | if exist('tl_check_ports','file')
      |     tl_check_ports(gcbh);
      | end
      settings: NameChangeFcn=|
      | if exist('rename_tlblock','file')==2,rename_tlblock(gcbh);end
      | if exist('tl_check_ports','file'), tl_check_ports(gcbh); end
      mask Help: eval(['if exist(''tl_online_help'',''file'') == 2, tl_online_help(''Topic'',''TL_Outport''),else, web([''jar:file:///'',matlabroot,''/help/toolbox/simulink/help.jar!/slref/' lower(get_param(gcbh,'Blocktype')) '.html''], ''-helpbrowser''),end'])
      mask Display: plot([0.2 0.35 NaN 0.65 0.8],[0 1 NaN 0 1]);
  gp_test : Outport  Port=7  PortDimensions=1  OutDataType=sfix(16)  OutScaling=2^0  mask(TL_Outport){data={'logdata',{'plotchannels',[]},'output',{'type','Bool'},'date',734178.39642236114}}
      settings: DeleteFcn=if exist('delete_tlblock','file')==2,delete_tlblock(gcbh);end  OpenFcn=if exist('tl_open_blockdlg','file')==2,tl_open_blockdlg(gcbh);else,open_system(gcbh,'parameter');end
      settings: CopyFcn=|
      | if exist('tl_reset_reviewflag','file')==2
      |     tl_reset_reviewflag(gcbh);
      | end
      | if exist('tl_check_ports','file')
      |     tl_check_ports(gcbh);
      | end
      settings: NameChangeFcn=|
      | if exist('rename_tlblock','file')==2,rename_tlblock(gcbh);end
      | if exist('tl_check_ports','file'), tl_check_ports(gcbh); end
      mask Help: eval(['if exist(''tl_online_help'',''file'') == 2, tl_online_help(''Topic'',''TL_Outport''),else, web([''jar:file:///'',matlabroot,''/help/toolbox/simulink/help.jar!/slref/' lower(get_param(gcbh,'Blocktype')) '.html''], ''-helpbrowser''),end'])
      mask Display: plot([0.2 0.35 NaN 0.65 0.8],[0 1 NaN 0 1]);
  ap_test : Outport  Port=8  PortDimensions=1  OutDataType=sfix(16)  OutScaling=2^0  mask(TL_Outport){data={'logdata',{'plotchannels',[]},'output',{'type','Bool'},'date',734178.39642181713}}
      settings: DeleteFcn=if exist('delete_tlblock','file')==2,delete_tlblock(gcbh);end  OpenFcn=if exist('tl_open_blockdlg','file')==2,tl_open_blockdlg(gcbh);else,open_system(gcbh,'parameter');end
      settings: CopyFcn=|
      | if exist('tl_reset_reviewflag','file')==2
      |     tl_reset_reviewflag(gcbh);
      | end
      | if exist('tl_check_ports','file')
      |     tl_check_ports(gcbh);
      | end
      settings: NameChangeFcn=|
      | if exist('rename_tlblock','file')==2,rename_tlblock(gcbh);end
      | if exist('tl_check_ports','file'), tl_check_ports(gcbh); end
      mask Help: eval(['if exist(''tl_online_help'',''file'') == 2, tl_online_help(''Topic'',''TL_Outport''),else, web([''jar:file:///'',matlabroot,''/help/toolbox/simulink/help.jar!/slref/' lower(get_param(gcbh,'Blocktype')) '.html''], ''-helpbrowser''),end'])
      mask Display: plot([0.2 0.35 NaN 0.65 0.8],[0 1 NaN 0 1]);
  flame_test : Outport  Port=9  PortDimensions=1  OutDataType=sfix(16)  OutScaling=2^0  mask(TL_Outport){data={'logdata',{'plotchannels',[]},'date',734178.39642108791}}
      settings: DeleteFcn=if exist('delete_tlblock','file')==2,delete_tlblock(gcbh);end  OpenFcn=if exist('tl_open_blockdlg','file')==2,tl_open_blockdlg(gcbh);else,open_system(gcbh,'parameter');end
      settings: CopyFcn=|
      | if exist('tl_reset_reviewflag','file')==2
      |     tl_reset_reviewflag(gcbh);
      | end
      | if exist('tl_check_ports','file')
      |     tl_check_ports(gcbh);
      | end
      settings: NameChangeFcn=|
      | if exist('rename_tlblock','file')==2,rename_tlblock(gcbh);end
      | if exist('tl_check_ports','file'), tl_check_ports(gcbh); end
      mask Help: eval(['if exist(''tl_online_help'',''file'') == 2, tl_online_help(''Topic'',''TL_Outport''),else, web([''jar:file:///'',matlabroot,''/help/toolbox/simulink/help.jar!/slref/' lower(get_param(gcbh,'Blocktype')) '.html''], ''-helpbrowser''),end'])
      mask Display: plot([0.2 0.35 NaN 0.65 0.8],[0 1 NaN 0 1]);
  wires:
  input_verification/6(Out6) -> flame_test/1
  input_verification/5(Out5) -> ap_test/1
  input_verification/4(Out4) -> gp_test/1
  fanspeedcontrol/1(fanspeed) -> fanspeed/1
  output_verification/3(Out3) -> ignition/1
  output_verification/2(Out2) -> y1/1
  output_verification/1(Out1) -> m1/1
  reg_ratio/1 -> fanspeedcontrol/2(reg_ratio)
  lockout_reset/1 -> lockcontroller/3(reset_in)
  fs_ignition/1 -> output_verification/3(In3)
  fs_y1/1 -> output_verification/2(In2)
  fs_m1/1 -> output_verification/1(In1)
  flame/1 -> input_verification/3(In3)
  ap/1 -> input_verification/2(In2)
  gp/1 -> input_verification/1(In1)
  clk/1 -> maincontroller/1(clk)
  tr/1 -> maincontroller/5(tr_in)
  pwron/1 -> maincontroller/4(pwron_in)
  input_verification/1(Out1) -> maincontroller/6(gp_on)
  input_verification/2(Out2) -> maincontroller/7(ap_on)
  input_verification/3(Out3) -> maincontroller/8(flame_on)
  maincontroller/1(m1_on) -> output_verification/4(In4)
  maincontroller/2(y1_on) -> output_verification/5(In5)
  maincontroller/3(ignition_on) -> output_verification/6(In6)
  input_verification/7(Out7) -> lockcontroller/2(srinplock)
  maincontroller/5(mainctrllock) -> lockcontroller/1(mainctrlock)
  output_verification/4(Out4) -> lockcontroller/4(sroutplock)
  lockcontroller/2(unlock) -> [unlock]
  maincontroller/4(stateno) -> fanspeedcontrol/1(stateno), statusdisp/1
  [unlock] -> maincontroller/2(unlock)
  [lock] -> maincontroller/3(lock)
  lockcontroller/1(lock) -> [lock], errordisp/1
